simulink model "wrench_observer"  (R2018b)
settings: Solver=VariableStepAuto  StartTime=0.0  StopTime=0.75  RelTol=1e-3
InitFcn:
  | %x_k1 = 0.00001*ones(36,1); % initialisation with initial state uncertainity
  | %P_k1 = 0.00001*ones(36); % initialisation with initial state uncertainity
values from neighbouring files (symbols this model uses):
  a_noise = 0    [parameter.m]
  alpha1 = pi/2    (= 1.57079632679)    [parameter.m]
  alpha2 = 0    [parameter.m]
  alpha3 = 0    [parameter.m]
  angular_noise = 0    [parameter.m]
  g = 9.81    [parameter.m]
  K_f_comm = 1    [parameter.m]
  K_I = [500*eye(3), zeros(3), zeros(3) ... (first row only)    [parameter.m]
  K_tau_comm = 1    [parameter.m]
  K_tau_man_comm = 1    [parameter.m]
  m = 3.9    [parameter.m]
  m_l1 = 0.3    [parameter.m]
  m_l2 = 0.35    [parameter.m]
  m_l3 = 0.35    [parameter.m]
  N_m = 1*diag([(p_noise/(3*noise_factor))^2 (p_noise/(3*noise_factor))^2 (p_noise/(3*noise_factor))^2 (a_noise/(3*noise_factor))^2 (a_noise/(3*noise_factor))^2 (a_noise/(3*noise_factor))^2 (angular_noise/(3*noise_factor))^2 (angular_noise/(3*noise_factor))^2 (angular_noise/(3*noise_factor))^2 (omega_noise/(3*noise_factor))^2 (omega_noise/(3*noise_factor))^2 (omega_noise/(3*noise_factor))^2 (theta_noise/( ...(+272 chars)    [parameter.m]
  N_p = diag(noise_factor_EKF)    [parameter.m]
  omega_dot_noise = 0    [parameter.m]
  omega_noise = 0    [parameter.m]
  p_L1_l1 = [p_L1_x_l1 p_L1_y_l1 p_L1_z_l1]'    [parameter.m]
  p_L2_l2 = [p_L2_x_l2 p_L2_y_l2 p_L2_z_l2]'    [parameter.m]
  p_L3_l3 = [p_L3_x_l3 p_L3_y_l3 p_L3_z_l3]'    [parameter.m]
  p_noise = 0    [parameter.m]
  R_B_L0 = [1 0 0;0 1 0; 0 0 1]    [parameter.m]
  T_delay = 0    [parameter.m]
  T_dis = 0.01    [parameter.m]
  theta_dot_dot_noise = 0    [parameter.m]
  theta_dot_noise = 0    [parameter.m]
  theta_noise = 0    [parameter.m]
  Ts = 1/250    (= 0.004)    [parameter.m]
  v_noise = 0    [parameter.m]
libraries: simulink x9, dspstat3 x2, dspinverses x1
(part 1 of 5)
settings Model: SimulationMode=accelerator  Creator=Marek  LastModifiedBy=Marek
settings OptimizationCC: EfficientMapNaN2IntZero=off
settings HardwareCC: TargetBitPerPointer=64  TargetBitPerSizeT=64  TargetBitPerPtrDiffT=64  TargetLongLongMode=on  TargetIntDivRoundTo=Zero  TargetEndianess=LittleEndian  TargetWordSize=64  TargetHWDeviceType=MATLAB Host  ProdEqTarget=off
settings CodeAppCC: MaxIdLength=128
settings GRTTargetCC: TargetLangStandard=C89/C90 (ANSI)  CombineOutputUpdateFcns=off  GRTInterface=on

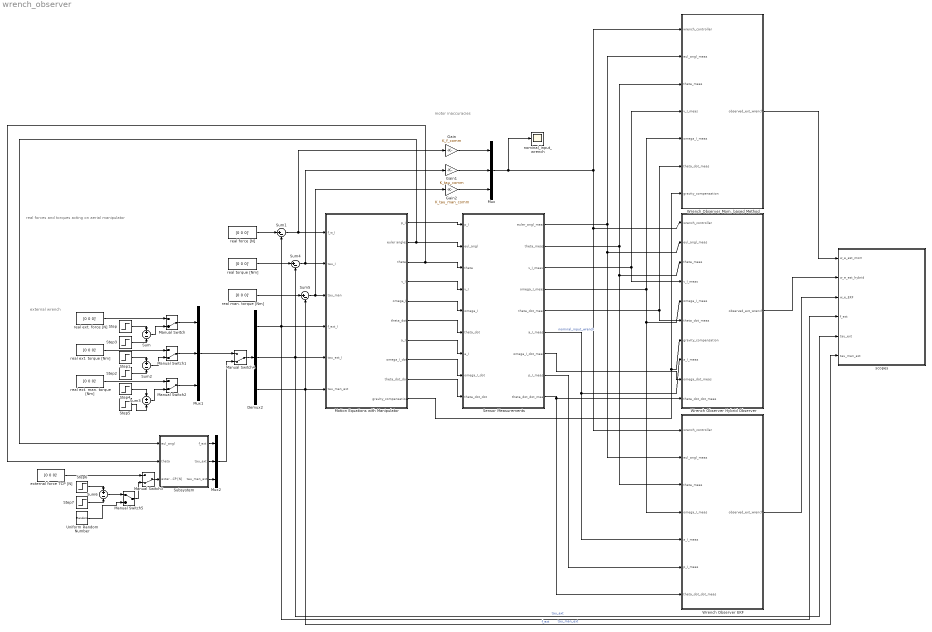
== system wrench_observer ==
  note: external wrench
  note: motor inaccuracies
  note: real forces and torques acting on aerial manipulator
  " external force TCP [N]" : Constant  Value=[0 0 0]'
  Demux2 : Demux  Outputs=3
  Gain : Gain  Gain=K_f_comm
  Gain1 : Gain  Gain=K_tau_comm
  Gain2 : Gain  Gain=K_tau_man_comm
  Manual Switch{,1..4} (5 alike) : ManualSwitch  CurrentSetting=0
  Manual Switch5 : ManualSwitch
  "Motion Equations with Manipulator " : Subsystem
  Mux : Mux  Inputs=3
  Mux1 : Mux  Inputs=3
  Mux2 : Mux  Inputs=3
  Sensor Measurements : Subsystem
  Step : Step  Time=0.2  Before=[0 0 0]'  After=[50 0 0]'  SampleTime=0
  Step1 : Step  Time=0.2  Before=[0 0 0]'  After=[0 100 0]'  SampleTime=0
  Step2 : Step  Time=0.7  Before=[0 0 0]'  After=[0 1 0]'  SampleTime=0
  Step3 : Step  Time=2.5  Before=[0 0 0]'  After=[50 0 0]'  SampleTime=0
  Step4 : Step  Time=0.2  Before=[0 0 0]'  After=[30 0 -45]'  SampleTime=0
  Step5 : Step  Time=0.7  Before=[0 0 0]'  After=[30 0 20]'  SampleTime=0
  Step6 : Step  Time=0.2  Before=[0 0 0]'  After=[50 0 -30]'  SampleTime=0
  Step7 : Step  Time=0.6  Before=[0 0 0]'  After=[50 0 -30]'  SampleTime=0
  Subsystem : Subsystem
  Sum{,2..3,6} (4 alike) : Sum  Inputs=+|-
  Sum1 : Sum  Inputs=|+-
  Sum4 : Sum  Inputs=|+-
  Sum5 : Sum  Inputs=|+-
  Uniform Random Number : UniformRandomNumber  Minimum=-50  Maximum=50  Seed=23  SampleTime=0.1
  Wrench Observer EKF : Subsystem
  Wrench Observer Hybrid Observer : Subsystem
  Wrench Observer Mom. based Method : Subsystem
  nominal_input_wrench : Scope
  real ext. force [N] : Constant  Value=[0 0 0]'
  real ext. man. torque [Nm] : Constant  Value=[0 0 0]'
  real ext. torque [Nm] : Constant  Value=[0 0 0]'
  real force [N] : Constant  Value=[0 0 0]'
  "real man. torque [Nm] " : Constant  Value=[0 0 0]'
  real torque [Nm] : Constant  Value=[0 0 0]'
  scopes : Subsystem
  wires:
  "Motion Equations with Manipulator "/1(p_I) -> Sensor Measurements/1(p_I)
  "Motion Equations with Manipulator "/2(euler angles) -> Subsystem/1(eul_angl), Sensor Measurements/2(eul_angl)
  "Motion Equations with Manipulator "/4(v_I) -> Sensor Measurements/4(v_I)
  "Motion Equations with Manipulator "/5(omega_I) -> Sensor Measurements/5(omega_I)
  "Motion Equations with Manipulator "/6(theta_dot) -> Sensor Measurements/6(theta_dot)
  "Motion Equations with Manipulator "/7(a_I) -> Sensor Measurements/7(a_I)
  "Motion Equations with Manipulator "/8(omega_I_dot) -> Sensor Measurements/8(omega_I_dot)
  "Motion Equations with Manipulator "/9(theta_dot_dot) -> Sensor Measurements/9(theta_dot_dot)
  Sum1/1 -> Gain/1, "Motion Equations with Manipulator "/1("f_w_I ")
  Sum5/1 -> Gain2/1, "Motion Equations with Manipulator "/3("tau_man ")
  Sum4/1 -> Gain1/1, "Motion Equations with Manipulator "/2(tau_I)
  Sensor Measurements/1(euler_angl_meas) -> Wrench Observer EKF/2(eul_angl_meas), Wrench Observer Hybrid Observer/2(eul_angl_meas), Wrench Observer Mom. based Method/2(eul_angl_meas)
  Sensor Measurements/2(theta_meas) -> Wrench Observer EKF/3(theta_meas), Wrench Observer Hybrid Observer/3(theta_meas), Wrench Observer Mom. based Method/3(theta_meas)
  Sensor Measurements/3(v_I_meas) -> Wrench Observer Hybrid Observer/4(v_I_meas), Wrench Observer Mom. based Method/4(v_I_meas)
  Sensor Measurements/4(omega_I_meas) -> Wrench Observer EKF/4(omega_I_meas), Wrench Observer Hybrid Observer/5(omega_I_meas), Wrench Observer Mom. based Method/5(omega_I_meas)
  Sensor Measurements/5(theta_dot_meas) -> Wrench Observer Hybrid Observer/6(theta_dot_meas), Wrench Observer Mom. based Method/6(theta_dot_meas)
  Sensor Measurements/6(a_I_meas) -> Wrench Observer Hybrid Observer/8(a_I_meas), Wrench Observer EKF/5(a_I_meas)
  Sensor Measurements/9(theta_dot_dot_meas) -> Wrench Observer Hybrid Observer/10(theta_dot_dot_meas), Wrench Observer EKF/7(theta_dot_dot_meas)
  Sensor Measurements/8(p_I_meas) -> Wrench Observer EKF/6(p_I_meas)
  Mux/1 -> nominal_input_wrench/1, Wrench Observer Mom. based Method/1(wrench_controller), Wrench Observer Hybrid Observer/1(wrench_controller), Wrench Observer EKF/1(wrench_controller)  "nominal_input_wrench"
  "Motion Equations with Manipulator "/10(gravity_compensation) -> Wrench Observer Hybrid Observer/7(gravity_compensation), Wrench Observer Mom. based Method/7(gravity_compensation)
  real ext. torque [Nm]/1 -> Manual Switch1/1
  real ext. man. torque [Nm]/1 -> Manual Switch2/1
  Step3/1 -> Sum/2
  Step/1 -> Sum/1
  Sum/1 -> Manual Switch/2
  Step2/1 -> Sum2/2
  Step1/1 -> Sum2/1
  Sum2/1 -> Manual Switch1/2
  Step5/1 -> Sum3/2
  Step4/1 -> Sum3/1
  Sum3/1 -> Manual Switch2/2
  real ext. force [N]/1 -> Manual Switch/1
  "Motion Equations with Manipulator "/3(theta) -> Sensor Measurements/3(theta), Subsystem/2(theta)
  Step6/1 -> Sum6/1
  Sum6/1 -> Manual Switch5/1
  Step7/1 -> Sum6/2
  Manual Switch3/1 -> Subsystem/3(external force TCP [N])
  Manual Switch/1 -> Mux1/1
  Manual Switch1/1 -> Mux1/2
  Manual Switch2/1 -> Mux1/3
  Demux2/1 -> scopes/4(f_ext), "Motion Equations with Manipulator "/4(f_ext_I), Sum1/2  "f_ext"
  Demux2/2 -> scopes/5(tau_ext), Sum4/2, "Motion Equations with Manipulator "/5(tau_ext_I)  "tau_ext"
  Demux2/3 -> scopes/6(tau_man_ext), Sum5/2, "Motion Equations with Manipulator "/6("tau_man_ext ")  "tau_man_ext"
  Mux1/1 -> Manual Switch4/1
  Subsystem/2(tau_ext) -> Mux2/2
  Subsystem/3(tau_man_ext) -> Mux2/3
  Subsystem/1(f_ext) -> Mux2/1
  Mux2/1 -> Manual Switch4/2
  Manual Switch4/1 -> Demux2/1
  Uniform Random Number/1 -> Manual Switch5/2
  Manual Switch5/1 -> Manual Switch3/2
  real force [N]/1 -> Sum1/1
  real torque [Nm]/1 -> Sum4/1
  "real man. torque [Nm] "/1 -> Sum5/1
  " external force TCP [N]"/1 -> Manual Switch3/1
  Gain/1 -> Mux/1
  Gain1/1 -> Mux/2
  Gain2/1 -> Mux/3
  Sensor Measurements/7(omega_I_dot_meas) -> Wrench Observer Hybrid Observer/9(omega_dot_meas)
  Wrench Observer Mom. based Method/1(observed_ext_wrench) -> scopes/1(w_e_est_mom)
  Wrench Observer Hybrid Observer/1(observed_ext_wrench) -> scopes/2(w_e_est_hybrid)
  Wrench Observer EKF/1(observed_ext_wrench) -> scopes/3(w_e_EKF)

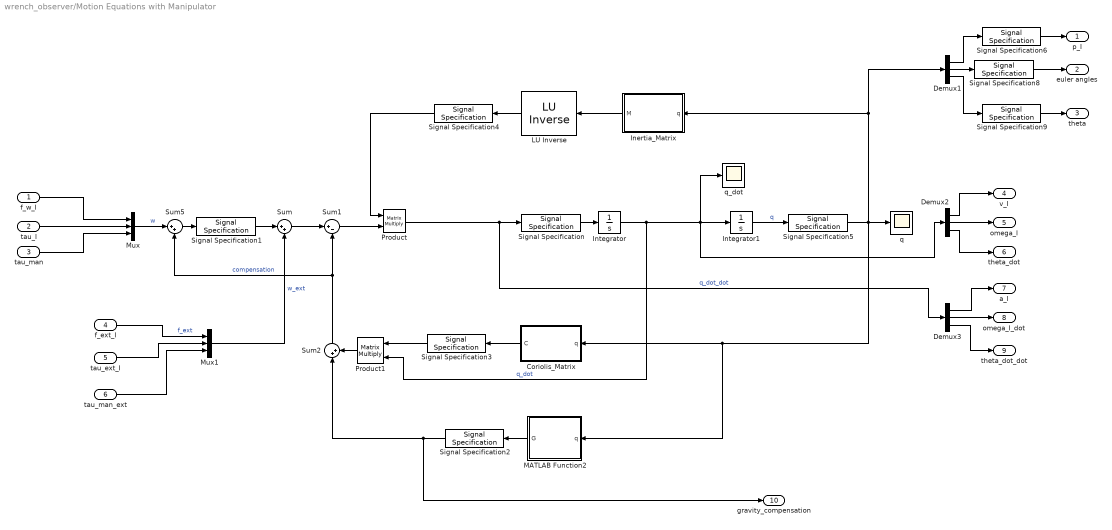
== system wrench_observer/Motion Equations with Manipulator  ==
  "f_w_I " : Inport
  tau_I : Inport  Port=2
  "tau_man " : Inport  Port=3
  f_ext_I : Inport  Port=4  PortDimensions=3
  tau_ext_I : Inport  Port=5  PortDimensions=3
  "tau_man_ext " : Inport  Port=6  PortDimensions=3
  " LU Inverse" : dspinverses/ LU Inverse
      settings: SourceProductName=DSP System Toolbox
  Coriolis_Matrix : Subsystem
  Demux1 : Demux  Outputs=3
  Demux2 : Demux  Outputs=3
  Demux3 : Demux  Outputs=3
  Inertia_Matrix : Subsystem
  Integrator : Integrator  InitialCondition=[0 0 0 0 0 0 0 0 0]'
  Integrator1 : Integrator  InitialCondition=[1 0.75 1 0.1 0.1 0.1 pi/3 pi/3 pi/3]'
  MATLAB Function2 : MATLAB Function  TreatAsAtomicUnit=on
  Mux : Mux  Inputs=3
  Mux1 : Mux  Inputs=3
  Product : Product  Multiplication=Matrix(*)  OutDataTypeStr=Inherit: Same as first input
  Product1 : Product  Multiplication=Matrix(*)
  Signal Specification{,1..2,5} (4 alike) : SignalSpecification  Dimensions=[9 1]
  Signal Specification3 : SignalSpecification  Dimensions=[9 9]
  Signal Specification4 : SignalSpecification  Dimensions=[9 9]
  Signal Specification6 : SignalSpecification  Dimensions=[3 1]
  Signal Specification8 : SignalSpecification  Dimensions=[3 1]
  Signal Specification9 : SignalSpecification  Dimensions=[3 1]
  Sum : Sum  Inputs=|++
  Sum1 : Sum  Inputs=|+-
  Sum2 : Sum  Inputs=|++
  Sum5 : Sum  Inputs=|++
  q : Scope
  q_dot : Scope
  p_I : Outport
  euler angles : Outport  Port=2
  theta : Outport  Port=3
  v_I : Outport  Port=4
  omega_I : Outport  Port=5
  theta_dot : Outport  Port=6
  a_I : Outport  Port=7
  omega_I_dot : Outport  Port=8
  theta_dot_dot : Outport  Port=9
  gravity_compensation : Outport  Port=10
  wires:
  "f_w_I "/1 -> Mux/1
  tau_I/1 -> Mux/2
  f_ext_I/1 -> Mux1/1  "f_ext"
  tau_ext_I/1 -> Mux1/2
  Mux/1 -> Sum5/1  "w"
  Sum/1 -> Sum1/1
  Sum2/1 -> Sum5/2, Sum1/2  "compensation"
  Integrator/1 -> q_dot/1, Demux2/1, Integrator1/1, Product1/2  "q_dot"
  Integrator1/1 -> Signal Specification5/1  "q"
  Sum1/1 -> Product/2
  Demux1/1 -> Signal Specification6/1
  Demux2/2 -> omega_I/1
  Demux1/3 -> Signal Specification9/1
  Demux2/1 -> v_I/1
  Demux2/3 -> theta_dot/1
  Demux3/1 -> a_I/1
  Demux3/2 -> omega_I_dot/1
  Demux3/3 -> theta_dot_dot/1
  Product1/1 -> Sum2/2
  "tau_man_ext "/1 -> Mux1/3
  "tau_man "/1 -> Mux/3
  Mux1/1 -> Sum/2  "w_ext"
  Signal Specification/1 -> Integrator/1
  Signal Specification1/1 -> Sum/1
  Signal Specification3/1 -> Product1/1
  " LU Inverse"/1 -> Signal Specification4/1
  Signal Specification4/1 -> Product/1
  Signal Specification5/1 -> Demux1/1, Inertia_Matrix/1(q), q/1, MATLAB Function2/1(q), Coriolis_Matrix/1(q)
  Demux1/2 -> Signal Specification8/1
  MATLAB Function2/1(G) -> Signal Specification2/1
  Inertia_Matrix/1(M) -> " LU Inverse"/1
  Coriolis_Matrix/1(C) -> Signal Specification3/1
  Signal Specification6/1 -> p_I/1
  Signal Specification8/1 -> euler angles/1
  Signal Specification9/1 -> theta/1
  Product/1 -> Demux3/1, Signal Specification/1  "q_dot_dot"
  Signal Specification2/1 -> gravity_compensation/1, Sum2/1
  Sum5/1 -> Signal Specification1/1

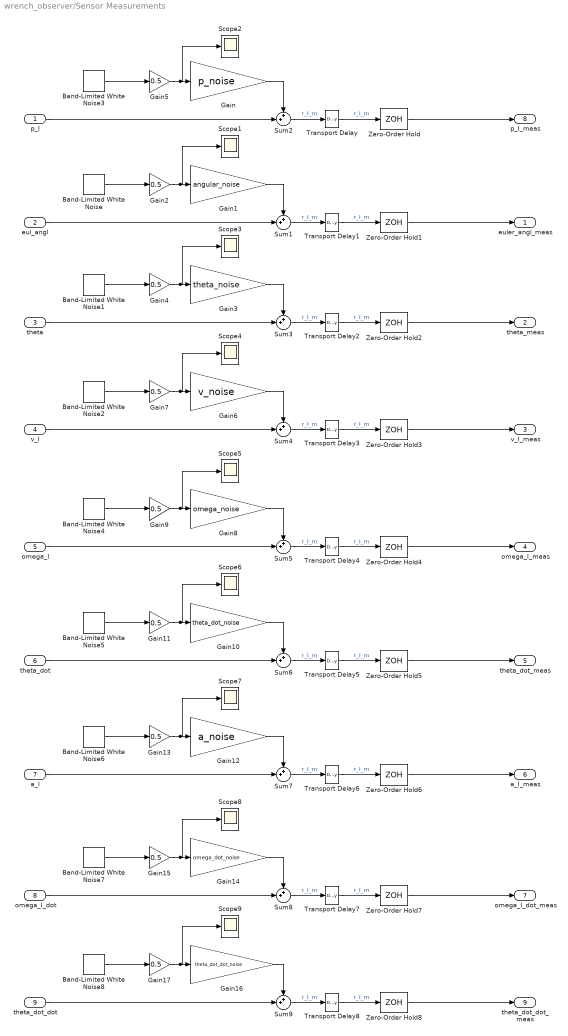
== system wrench_observer/Sensor Measurements ==
  p_I : Inport
  eul_angl : Inport  Port=2
  theta : Inport  Port=3
  v_I : Inport  Port=4
  omega_I : Inport  Port=5
  theta_dot : Inport  Port=6
  a_I : Inport  Port=7
  omega_I_dot : Inport  Port=8
  theta_dot_dot : Inport  Port=9
  Band-Limited White Noise : simulink/Sources/Band-Limited White Noise  Cov=noise_power  Ts=Ts  seed=[23341 2342 3453]'
  Band-Limited White Noise1 : simulink/Sources/Band-Limited White Noise  Cov=noise_power  Ts=Ts  seed=[23346 234 2345]'
  Band-Limited White Noise2 : simulink/Sources/Band-Limited White Noise  Cov=noise_power  Ts=Ts  seed=[233412 1234435 23]'
  Band-Limited White Noise3 : simulink/Sources/Band-Limited White Noise  Cov=noise_power  Ts=Ts  seed=[22352; 29655; 12541]  VectorParams1D=off
  Band-Limited White Noise4 : simulink/Sources/Band-Limited White Noise  Cov=noise_power  Ts=Ts  seed=[23341 34512 234345]'
  Band-Limited White Noise5 : simulink/Sources/Band-Limited White Noise  Cov=noise_power  Ts=Ts  seed=[23341 2345 231]'
  Band-Limited White Noise6 : simulink/Sources/Band-Limited White Noise  Cov=noise_power  Ts=Ts  seed=[235 3451 4352]'
  Band-Limited White Noise7 : simulink/Sources/Band-Limited White Noise  Cov=noise_power  Ts=Ts  seed=[3462 56735 1234]'
  Band-Limited White Noise8 : simulink/Sources/Band-Limited White Noise  Cov=noise_power  Ts=Ts  seed=[23341 2345 1234]'
  Gain : Gain  Gain=p_noise
  Gain1 : Gain  Gain=angular_noise
  Gain10 : Gain  Gain=theta_dot_noise
  Gain{2,4..5,7,9,11,13,15,17} (9 alike) : Gain  Gain=0.5
  Gain12 : Gain  Gain=a_noise
  Gain14 : Gain  Gain=omega_dot_noise
  Gain16 : Gain  Gain=theta_dot_dot_noise
  Gain3 : Gain  Gain=theta_noise
  Gain6 : Gain  Gain=v_noise
  Gain8 : Gain  Gain=omega_noise
  Scope{1..9} (9 alike) : Scope
  Sum{1..9} (9 alike) : Sum  Inputs=++|
  Transport Delay{,1..8} (9 alike) : TransportDelay  DelayTime=T_delay  InitialOutput=[0;0;0]
  Zero-Order Hold{,1..8} (9 alike) : ZeroOrderHold  SampleTime=0.02
  euler_angl_meas : Outport
  theta_meas : Outport  Port=2
  v_I_meas : Outport  Port=3
  omega_I_meas : Outport  Port=4
  theta_dot_meas : Outport  Port=5
  a_I_meas : Outport  Port=6
  omega_I_dot_meas : Outport  Port=7
  p_I_meas : Outport  Port=8
  theta_dot_dot_meas : Outport  Port=9
  wires:
  Gain5/1 -> Scope2/1, Gain/1
  Band-Limited White Noise3/1 -> Gain5/1
  Sum2/1 -> Transport Delay/1  "r_I_m"
  Gain/1 -> Sum2/1
  Transport Delay/1 -> Zero-Order Hold/1  "r_I_m"
  p_I/1 -> Sum2/2
  Zero-Order Hold/1 -> p_I_meas/1
  Transport Delay1/1 -> Zero-Order Hold1/1  "r_I_m"
  Sum1/1 -> Transport Delay1/1  "r_I_m"
  Band-Limited White Noise/1 -> Gain2/1
  Gain1/1 -> Sum1/1
  eul_angl/1 -> Sum1/2
  Gain2/1 -> Scope1/1, Gain1/1
  Zero-Order Hold1/1 -> euler_angl_meas/1
  Band-Limited White Noise1/1 -> Gain4/1
  Gain4/1 -> Scope3/1, Gain3/1
  Sum3/1 -> Transport Delay2/1  "r_I_m"
  Gain3/1 -> Sum3/1
  Zero-Order Hold2/1 -> theta_meas/1
  Transport Delay2/1 -> Zero-Order Hold2/1  "r_I_m"
  theta/1 -> Sum3/2
  Band-Limited White Noise2/1 -> Gain7/1
  Gain7/1 -> Scope4/1, Gain6/1
  Sum4/1 -> Transport Delay3/1  "r_I_m"
  Gain6/1 -> Sum4/1
  Zero-Order Hold3/1 -> v_I_meas/1
  Transport Delay3/1 -> Zero-Order Hold3/1  "r_I_m"
  v_I/1 -> Sum4/2
  Band-Limited White Noise4/1 -> Gain9/1
  Gain9/1 -> Scope5/1, Gain8/1
  Sum5/1 -> Transport Delay4/1  "r_I_m"
  Gain8/1 -> Sum5/1
  Zero-Order Hold4/1 -> omega_I_meas/1
  Transport Delay4/1 -> Zero-Order Hold4/1  "r_I_m"
  omega_I/1 -> Sum5/2
  Band-Limited White Noise5/1 -> Gain11/1
  Gain11/1 -> Scope6/1, Gain10/1
  Sum6/1 -> Transport Delay5/1  "r_I_m"
  Gain10/1 -> Sum6/1
  Zero-Order Hold5/1 -> theta_dot_meas/1
  Transport Delay5/1 -> Zero-Order Hold5/1  "r_I_m"
  theta_dot/1 -> Sum6/2
  Band-Limited White Noise6/1 -> Gain13/1
  Gain13/1 -> Scope7/1, Gain12/1
  Sum7/1 -> Transport Delay6/1  "r_I_m"
  Gain12/1 -> Sum7/1
  Zero-Order Hold6/1 -> a_I_meas/1
  Transport Delay6/1 -> Zero-Order Hold6/1  "r_I_m"
  a_I/1 -> Sum7/2
  Band-Limited White Noise7/1 -> Gain15/1
  Gain15/1 -> Scope8/1, Gain14/1
  Sum8/1 -> Transport Delay7/1  "r_I_m"
  Gain14/1 -> Sum8/1
  Zero-Order Hold7/1 -> omega_I_dot_meas/1
  Transport Delay7/1 -> Zero-Order Hold7/1  "r_I_m"
  omega_I_dot/1 -> Sum8/2
  Band-Limited White Noise8/1 -> Gain17/1
  Gain17/1 -> Scope9/1, Gain16/1
  Sum9/1 -> Transport Delay8/1  "r_I_m"
  Gain16/1 -> Sum9/1
  Zero-Order Hold8/1 -> theta_dot_dot_meas/1
  Transport Delay8/1 -> Zero-Order Hold8/1  "r_I_m"
  theta_dot_dot/1 -> Sum9/2

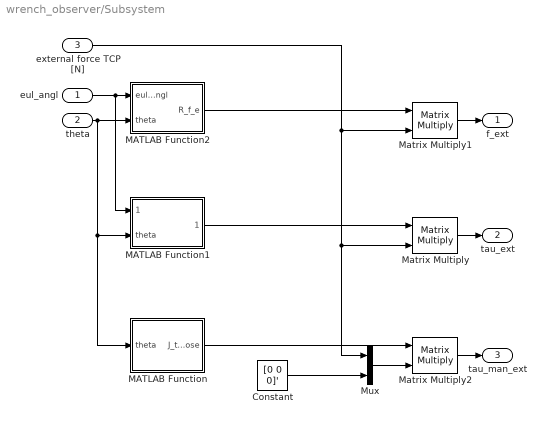
== system wrench_observer/Subsystem ==
  eul_angl : Inport
  theta : Inport  Port=2
  external force TCP [N] : Inport  Port=3
  Constant : Constant  Value=[0 0 0]'
  MATLAB Function : MATLAB Function  TreatAsAtomicUnit=on
  MATLAB Function1 : MATLAB Function  TreatAsAtomicUnit=on
  MATLAB Function2 : MATLAB Function  TreatAsAtomicUnit=on
  Matrix Multiply : Product  Multiplication=Matrix(*)
  Matrix Multiply1 : Product  Multiplication=Matrix(*)
  Matrix Multiply2 : Product  Multiplication=Matrix(*)
  Mux : Mux  Inputs=2
  f_ext : Outport
  tau_ext : Outport  Port=2
  tau_man_ext : Outport  Port=3
  wires:
  Matrix Multiply/1 -> tau_ext/1
  external force TCP [N]/1 -> Mux/1, Matrix Multiply/2, Matrix Multiply1/2
  Matrix Multiply2/1 -> tau_man_ext/1
  MATLAB Function/1(J_transpose) -> Matrix Multiply2/1
  Matrix Multiply1/1 -> f_ext/1
  MATLAB Function2/1(R_f_e) -> Matrix Multiply1/1
  MATLAB Function1/1(R_tau_e) -> Matrix Multiply/1
  eul_angl/1 -> MATLAB Function1/1(eul_angl), MATLAB Function2/1(eul_angl)
  theta/1 -> MATLAB Function1/2(theta), MATLAB Function/1(theta), MATLAB Function2/2(theta)
  Mux/1 -> Matrix Multiply2/2
  Constant/1 -> Mux/2

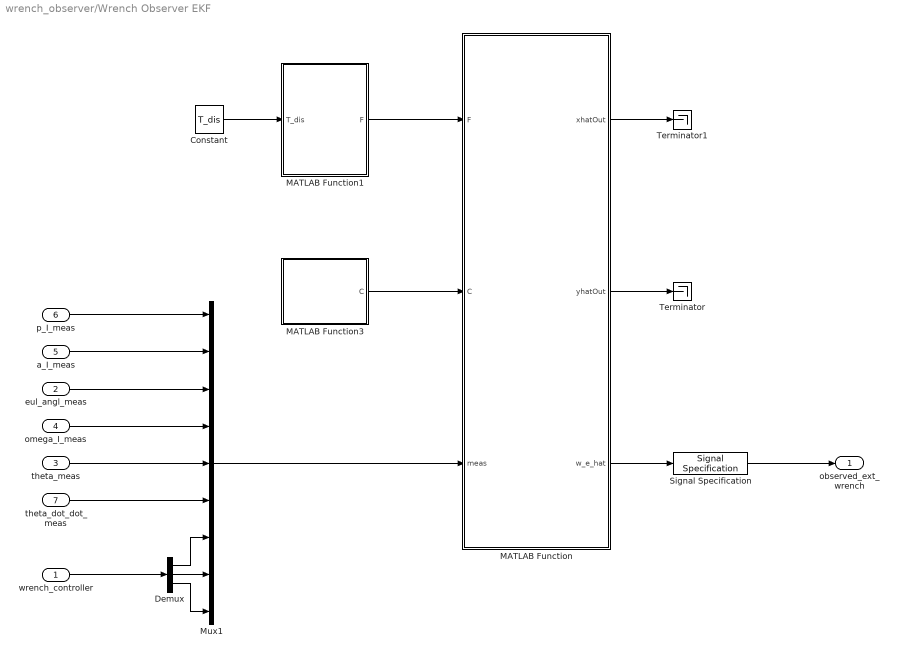
== system wrench_observer/Wrench Observer EKF ==
  wrench_controller : Inport
  eul_angl_meas : Inport  Port=2
  theta_meas : Inport  Port=3
  omega_I_meas : Inport  Port=4
  a_I_meas : Inport  Port=5
  p_I_meas : Inport  Port=6
  theta_dot_dot_meas : Inport  Port=7
  Constant : Constant  Value=T_dis
  Demux : Demux  Outputs=3
  MATLAB Function : MATLAB Function  InitFcn=|  TreatAsAtomicUnit=on
      | %x_k1 = [1 0.75 1 0 0 0 pi/4 pi/4 pi/4 0 0 0 pi/3 pi/3 pi/3 0 0 0 0 0 0 0 0 0 0 0 0 0 0 0 0 0 0 0 0 0]' 
      | %P_k1 = 0.0*ones(36); % initialisation with initial state uncertainity
      | %x_k_ = zeros(36,1);
      | %P_k_ = zeros(36);
      | %x_k = zeros(36,1);
      | %P_k = zeros(36);
  MATLAB Function1 : MATLAB Function  TreatAsAtomicUnit=on
  MATLAB Function3 : MATLAB Function  TreatAsAtomicUnit=on
  Mux1 : Mux  Inputs=9
  Signal Specification : SignalSpecification  Dimensions=[9 1]
  Terminator : Terminator
  Terminator1 : Terminator
  observed_ext_wrench : Outport
  wires:
  theta_dot_dot_meas/1 -> Mux1/6
  MATLAB Function/3(w_e_hat) -> Signal Specification/1
  Constant/1 -> MATLAB Function1/1(T_dis)
  MATLAB Function3/1(C) -> MATLAB Function/2(C)
  p_I_meas/1 -> Mux1/1
  a_I_meas/1 -> Mux1/2
  eul_angl_meas/1 -> Mux1/3
  omega_I_meas/1 -> Mux1/4
  theta_meas/1 -> Mux1/5
  MATLAB Function1/1(F) -> MATLAB Function/1(F)
  Demux/1 -> Mux1/7
  Demux/2 -> Mux1/8
  Demux/3 -> Mux1/9
  wrench_controller/1 -> Demux/1
  Mux1/1 -> MATLAB Function/3(meas)
  MATLAB Function/2(yhatOut) -> Terminator/1
  MATLAB Function/1(xhatOut) -> Terminator1/1
  Signal Specification/1 -> observed_ext_wrench/1

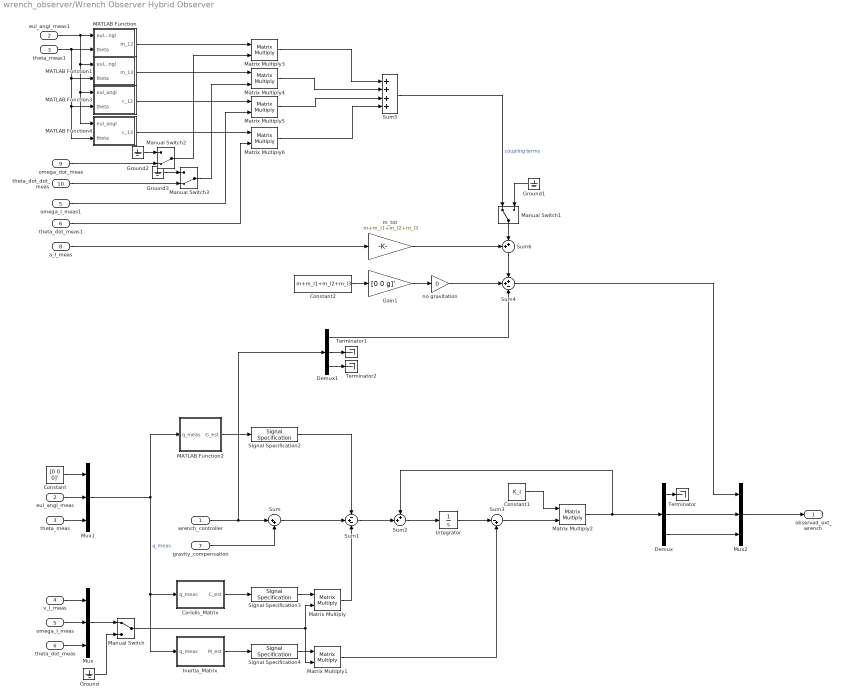
== system wrench_observer/Wrench Observer Hybrid Observer ==
  wrench_controller : Inport
  eul_angl_meas : Inport  Port=2
  theta_meas : Inport  Port=3
  v_I_meas : Inport  Port=4
  omega_I_meas : Inport  Port=5
  theta_dot_meas : Inport  Port=6
  gravity_compensation : Inport  Port=7
  a_I_meas : Inport  Port=8
  omega_dot_meas : Inport  Port=9
  theta_dot_dot_meas : Inport  Port=10
  Constant : Constant  Value=[0 0 0]'
  Constant1 : Constant  Value=K_I
  Constant2 : Constant  Value=m+m_l1+m_l2+m_l3
  Coriolis_Matrix : Subsystem
  Demux : Demux  Outputs=3
  Demux1 : Demux  Outputs=3
  Gain1 : Gain  Gain=[0 0 g]'
  Ground{,1..3} (4 alike) : Ground
  Inertia_Matrix : Subsystem
  Integrator : Integrator
  MATLAB Function : MATLAB Function  TreatAsAtomicUnit=on
  MATLAB Function1 : MATLAB Function  TreatAsAtomicUnit=on
  MATLAB Function2 : MATLAB Function  TreatAsAtomicUnit=on
  MATLAB Function3 : MATLAB Function  TreatAsAtomicUnit=on
  MATLAB Function4 : MATLAB Function  TreatAsAtomicUnit=on
  Manual Switch : ManualSwitch
  Manual Switch1 : ManualSwitch
  Manual Switch2 : ManualSwitch  CurrentSetting=0
  Manual Switch3 : ManualSwitch  CurrentSetting=0
  Matrix Multiply{,1..6} (7 alike) : Product  Multiplication=Matrix(*)
  Mux : Mux  Inputs=3
  Mux1 : Mux  Inputs=3
  Mux2 : Mux  Inputs=3
  Signal Specification2 : SignalSpecification  Dimensions=[9 1]
  Signal Specification3 : SignalSpecification  Dimensions=[9 9]
  Signal Specification4 : SignalSpecification  Dimensions=[9 9]
  Sum : Sum  Inputs=|++
  Sum1 : Sum  Inputs=-+-
  Sum2 : Sum  Inputs=++|
  Sum3 : Sum  Inputs=|-+
  Sum4 : Sum  Inputs=++-
  Sum5 : Sum  Inputs=++++
  Sum6 : Sum  Inputs=++|
  Terminator : Terminator
  Terminator1 : Terminator
  Terminator2 : Terminator
  eul_angl_meas1 : InportShadow  Port=2
  m_tot : Gain  Gain=m+m_l1+m_l2+m_l3
  no gravitation : Gain  Gain=0
  omega_I_meas1 : InportShadow  Port=5
  theta_dot_meas1 : InportShadow  Port=6
  theta_meas1 : InportShadow  Port=3
  observed_ext_wrench : Outport
  wires:
  wrench_controller/1 -> Demux1/1, Sum/1
  Signal Specification2/1 -> Sum1/1
  MATLAB Function2/1(G_est) -> Signal Specification2/1
  Sum/1 -> Sum1/2
  Sum1/1 -> Sum2/2
  Integrator/1 -> Sum3/1
  Inertia_Matrix/1(M_est) -> Signal Specification4/1
  Sum3/1 -> Matrix Multiply2/2
  Matrix Multiply2/1 -> Demux/1, Sum2/1
  Coriolis_Matrix/1(C_est) -> Signal Specification3/1
  omega_I_meas/1 -> Mux/2
  theta_dot_meas/1 -> Mux/3
  v_I_meas/1 -> Mux/1
  Signal Specification3/1 -> Matrix Multiply/1
  Manual Switch/1 -> Matrix Multiply/2, Matrix Multiply1/2
  Signal Specification4/1 -> Matrix Multiply1/1
  theta_meas/1 -> Mux1/3
  eul_angl_meas/1 -> Mux1/2
  Constant/1 -> Mux1/1
  Mux1/1 -> MATLAB Function2/1(q_meas), Inertia_Matrix/1(q_meas), Coriolis_Matrix/1(q_meas)  "q_meas"
  Matrix Multiply/1 -> Sum1/3
  Matrix Multiply1/1 -> Sum3/2
  Constant1/1 -> Matrix Multiply2/1
  gravity_compensation/1 -> Sum/2
  Demux/2 -> Mux2/2
  Demux/3 -> Mux2/3
  Mux2/1 -> observed_ext_wrench/1
  Demux/1 -> Terminator/1
  a_I_meas/1 -> m_tot/1
  Constant2/1 -> Gain1/1
  Sum4/1 -> Mux2/1
  Mux/1 -> Manual Switch/1
  Ground/1 -> Manual Switch/2
  Demux1/1 -> Sum4/3
  Demux1/2 -> Terminator1/1
  Demux1/3 -> Terminator2/1
  Sum2/1 -> Integrator/1
  Gain1/1 -> no gravitation/1
  no gravitation/1 -> Sum4/2
  eul_angl_meas1/1 -> MATLAB Function1/1(eul_angl), MATLAB Function3/1(eul_angl), MATLAB Function4/1(eul_angl), MATLAB Function/1(eul_angl)
  theta_meas1/1 -> MATLAB Function1/2(theta), MATLAB Function3/2(theta), MATLAB Function4/2(theta), MATLAB Function/2(theta)
  MATLAB Function/1(m_12) -> Matrix Multiply3/1
  MATLAB Function1/1(m_13) -> Matrix Multiply4/1
  MATLAB Function3/1(c_12) -> Matrix Multiply5/1
  MATLAB Function4/1(c_13) -> Matrix Multiply6/1
  omega_I_meas1/1 -> Matrix Multiply5/2
  theta_dot_meas1/1 -> Matrix Multiply6/2
  Matrix Multiply3/1 -> Sum5/1
  Matrix Multiply4/1 -> Sum5/2
  Matrix Multiply5/1 -> Sum5/3
  Matrix Multiply6/1 -> Sum5/4
  m_tot/1 -> Sum6/1
  Sum5/1 -> Manual Switch1/1  "coupling terms"
  Sum6/1 -> Sum4/1
  Manual Switch1/1 -> Sum6/2
  Ground1/1 -> Manual Switch1/2
  omega_dot_meas/1 -> Manual Switch2/2
  theta_dot_dot_meas/1 -> Manual Switch3/2
  Manual Switch3/1 -> Matrix Multiply4/2
  Manual Switch2/1 -> Matrix Multiply3/2
  Ground2/1 -> Manual Switch2/1
  Ground3/1 -> Manual Switch3/1

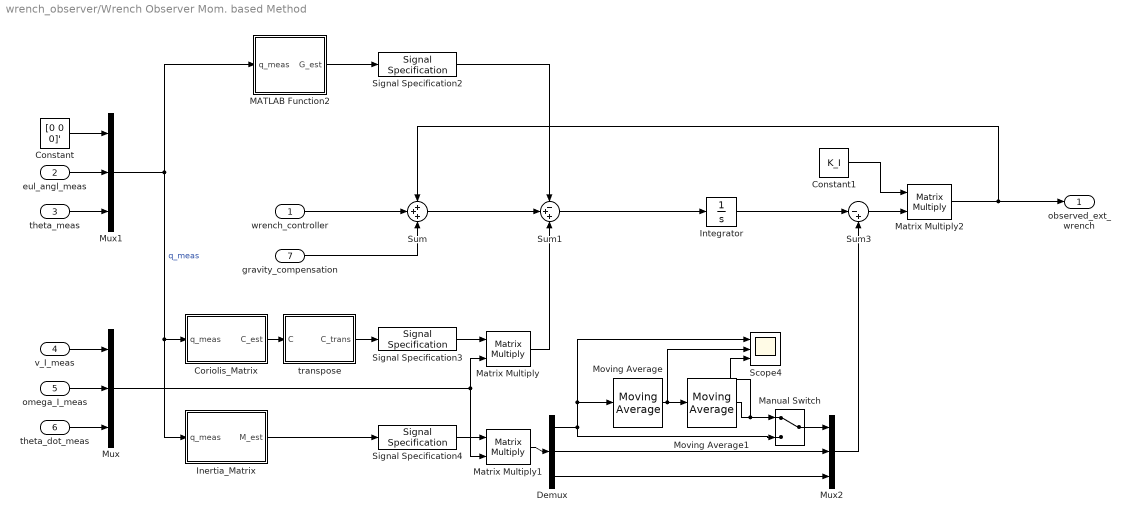
== system wrench_observer/Wrench Observer Mom. based Method ==
  wrench_controller : Inport
  eul_angl_meas : Inport  Port=2
  theta_meas : Inport  Port=3
  v_I_meas : Inport  Port=4
  omega_I_meas : Inport  Port=5
  theta_dot_meas : Inport  Port=6
  gravity_compensation : Inport  Port=7
  Constant : Constant  Value=[0 0 0]'
  Constant1 : Constant  Value=K_I
  Coriolis_Matrix : Subsystem
  Demux : Demux  Outputs=3
  Inertia_Matrix : Subsystem
  Integrator : Integrator
  MATLAB Function2 : MATLAB Function  TreatAsAtomicUnit=on
  Manual Switch : ManualSwitch
  Matrix Multiply : Product  Multiplication=Matrix(*)
  Matrix Multiply1 : Product  Multiplication=Matrix(*)
  Matrix Multiply2 : Product  Multiplication=Matrix(*)
  Moving Average : dspstat3/Moving Average  Method=Sliding window  ForgettingFactorPort=off  SpecifyWindowLength=on  WindowLength=10  ForgettingFactor=0.9  SimulateUsing=Interpreted execution
  Moving Average1 : dspstat3/Moving Average  Method=Sliding window  ForgettingFactorPort=off  SpecifyWindowLength=on  WindowLength=10  ForgettingFactor=0.9  SimulateUsing=Interpreted execution
  Mux : Mux  Inputs=3
  Mux1 : Mux  Inputs=3
  Mux2 : Mux  Inputs=3
  Scope4 : Scope  NumInputPorts=3
  Signal Specification2 : SignalSpecification  Dimensions=[9 1]
  Signal Specification3 : SignalSpecification  Dimensions=[9 9]
  Signal Specification4 : SignalSpecification  Dimensions=[9 9]
  Sum : Sum  Inputs=+++
  Sum1 : Sum  Inputs=-++
  Sum3 : Sum  Inputs=|-+
  transpose : MATLAB Function  TreatAsAtomicUnit=on
  observed_ext_wrench : Outport
  wires:
  wrench_controller/1 -> Sum/2
  Signal Specification2/1 -> Sum1/1
  MATLAB Function2/1(G_est) -> Signal Specification2/1
  Sum/1 -> Sum1/2
  Sum1/1 -> Integrator/1
  Integrator/1 -> Sum3/1
  Inertia_Matrix/1(M_est) -> Signal Specification4/1
  Sum3/1 -> Matrix Multiply2/2
  Matrix Multiply2/1 -> observed_ext_wrench/1, Sum/1
  omega_I_meas/1 -> Mux/2
  theta_dot_meas/1 -> Mux/3
  Signal Specification3/1 -> Matrix Multiply/1
  Mux/1 -> Matrix Multiply1/2, Matrix Multiply/2
  Signal Specification4/1 -> Matrix Multiply1/1
  theta_meas/1 -> Mux1/3
  eul_angl_meas/1 -> Mux1/2
  Constant/1 -> Mux1/1
  Mux1/1 -> MATLAB Function2/1(q_meas), Inertia_Matrix/1(q_meas), Coriolis_Matrix/1(q_meas)  "q_meas"
  Matrix Multiply/1 -> Sum1/3
  Constant1/1 -> Matrix Multiply2/1
  gravity_compensation/1 -> Sum/3
  v_I_meas/1 -> Mux/1
  Demux/3 -> Mux2/3
  Matrix Multiply1/1 -> Demux/1
  Demux/2 -> Mux2/2
  Mux2/1 -> Sum3/2
  Demux/1 -> Manual Switch/2, Scope4/1, Moving Average/1
  Moving Average/1 -> Scope4/2, Moving Average1/1
  Moving Average1/1 -> Scope4/3, Manual Switch/1
  Coriolis_Matrix/1(C_est) -> transpose/1(C)
  transpose/1(C_trans) -> Signal Specification3/1
  Manual Switch/1 -> Mux2/1

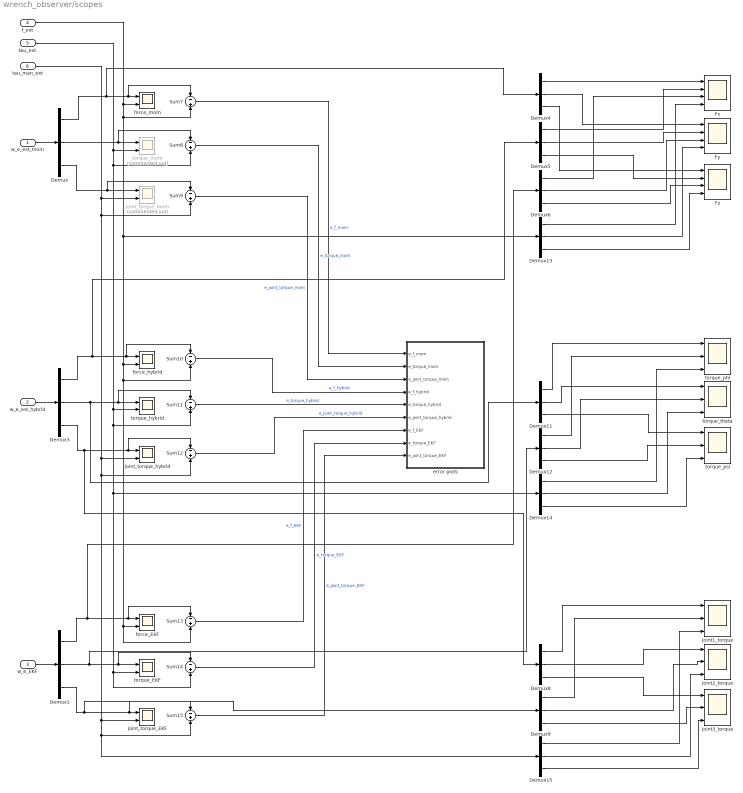
== system wrench_observer/scopes ==
  w_e_est_mom : Inport
  w_e_est_hybrid : Inport  Port=2
  w_e_EKF : Inport  Port=3
  f_ext : Inport  Port=4
  tau_ext : Inport  Port=5
  tau_man_ext : Inport  Port=6
  Demux{,1,3..6,8..9,11..15} (13 alike) : Demux  Outputs=3
  Fx : Scope  NumInputPorts=4
  Fy : Scope  NumInputPorts=4
  Fz : Scope  NumInputPorts=4
  Sum{7..15} (9 alike) : Sum  Inputs=-|+
  error plots : Subsystem
  force_EKF : Scope  NumInputPorts=2
  force_hybrid : Scope  NumInputPorts=2
  force_mom : Scope  NumInputPorts=2
  joint1_torque : Scope  NumInputPorts=3
  joint2_torque : Scope  NumInputPorts=3
  joint3_torque : Scope  NumInputPorts=3
  joint_torque_EKF : Scope  NumInputPorts=2
  joint_torque_hybrid : Scope  NumInputPorts=2
  joint_torque_mom : Scope  Commented=on  NumInputPorts=2
  torque_EKF : Scope  NumInputPorts=2
  torque_hybrid : Scope  NumInputPorts=2
  torque_mom : Scope  Commented=on  NumInputPorts=2
  torque_phi : Scope  NumInputPorts=3
  torque_psi : Scope  NumInputPorts=3
  torque_theta : Scope  NumInputPorts=3
  wires:
  Sum9/1 -> error plots/3(e_joint_torque_mom)  "e_joint_torque_mom"
  Demux3/3 -> Demux8/1, Sum12/1, joint_torque_hybrid/1
  Demux6/2 -> Fy/3
  tau_man_ext/1 -> Demux15/1, Sum15/2, joint_torque_EKF/2, Sum12/2, joint_torque_hybrid/2, Sum9/2, joint_torque_mom/2
  Demux/2 -> torque_mom/1, Sum8/1
  Demux3/1 -> Demux5/1, Sum10/1, force_hybrid/1
  Demux/1 -> Demux4/1, Sum7/1, force_mom/1
  f_ext/1 -> Sum13/2, force_EKF/2, Sum10/2, force_hybrid/2, Demux13/1, Sum7/2, force_mom/2
  tau_ext/1 -> Sum14/2, torque_EKF/2, Demux14/1, Sum11/2, torque_hybrid/2, Sum8/2, torque_mom/2
  Sum10/1 -> error plots/4(e_f_hybrid)  "e_f_hybrid"
  Demux12/1 -> torque_phi/2
  Demux/3 -> joint_torque_mom/1, Sum9/1
  Demux3/2 -> Demux11/1, Sum11/1, torque_hybrid/1
  Demux14/2 -> torque_theta/3
  Demux1/2 -> Demux12/1, Sum14/1, torque_EKF/1
  Demux1/1 -> Demux6/1, Sum13/1, force_EKF/1
  Demux6/1 -> Fx/3
  Demux4/1 -> Fx/1
  Demux5/1 -> Fx/2
  Demux8/1 -> joint1_torque/1
  Demux6/3 -> Fz/3
  Sum15/1 -> error plots/9(e_joint_torque_EKF)  "e_joint_torque_EKF"
  Demux4/2 -> Fy/1
  Demux1/3 -> Demux9/1, Sum15/1, joint_torque_EKF/1
  Demux15/2 -> joint2_torque/3
  Demux5/3 -> Fz/2
  Demux9/1 -> joint1_torque/2
  Demux4/3 -> Fz/1
  Demux11/2 -> torque_theta/1
  Sum7/1 -> error plots/1(e_f_mom)  "e_f_mom"
  Demux15/1 -> joint1_torque/3
  Demux5/2 -> Fy/2
  w_e_est_mom/1 -> Demux/1
  Demux13/2 -> Fy/4
  Sum14/1 -> error plots/8(e_torque_EKF)  "e_torque_EKF"
  Sum12/1 -> error plots/6(e_joint_torque_hybrid)  "e_joint_torque_hybrid"
  Demux13/3 -> Fz/4
  Demux12/2 -> torque_theta/2
  Demux14/1 -> torque_phi/3
  Demux8/3 -> joint3_torque/1
  Demux11/1 -> torque_phi/1
  Demux11/3 -> torque_psi/1
  Demux15/3 -> joint3_torque/3
  Demux9/2 -> joint2_torque/2
  Sum11/1 -> error plots/5(e_torque_hybrid)  "e_torque_hybrid"
  Sum13/1 -> error plots/7(e_f_EKF)  "e_f_EKF"
  Demux8/2 -> joint2_torque/1
  Demux9/3 -> joint3_torque/2
  Demux13/1 -> Fx/4
  Demux14/3 -> torque_psi/3
  Demux12/3 -> torque_psi/2
  Sum8/1 -> error plots/2(e_torque_mom)  "e_torque_mom"
  w_e_EKF/1 -> Demux1/1
  w_e_est_hybrid/1 -> Demux3/1

== system wrench_observer/Motion Equations with Manipulator /Coriolis_Matrix ==
  q : Inport
  Coriolis_Matrix_simplified : Subsystem
  Demux : Demux  Outputs=9
  Terminator : Terminator
  Terminator1 : Terminator
  Terminator2 : Terminator
  C : Outport
  wires:
  Demux/1 -> Terminator/1
  Demux/2 -> Terminator1/1
  Demux/6 -> Coriolis_Matrix_simplified/3(psi)
  Demux/5 -> Coriolis_Matrix_simplified/2(the)
  Demux/7 -> Coriolis_Matrix_simplified/4(theta1)
  Demux/8 -> Coriolis_Matrix_simplified/5(theta2)
  Demux/4 -> Coriolis_Matrix_simplified/1(phi)
  Demux/9 -> Coriolis_Matrix_simplified/6(theta3)
  Demux/3 -> Terminator2/1
  Coriolis_Matrix_simplified/1(C) -> C/1
  q/1 -> Demux/1

== system wrench_observer/Motion Equations with Manipulator /Inertia_Matrix ==
  q : Inport
  Demux4 : Demux  Outputs=9
  S-Function Builder : S-Function  InitFcn=try, set_param(gcb,'FunctionName','Inertia_Matrix_simplified'), end  FunctionName=Inertia_Matrix_simplified  SFunctionModules=Inertia_Matrix_simplified_wrapper Inertia_Matrix Inertia_Matrix_initialize Inertia_Matrix_terminate rt_nonfinite rtGetInf rtGetNaN  SFunctionDeploymentMode=off  EnableBusSupport=off  mask(S-Function Builder){}
      mask help: Simulink:masks:SFunctionBuilder_MD
      mask init:
      | val = [[.9  0.75 0.75 1 1 .9 .9 1]',[1 1 0.75 0.75 .9 .9 1 .9]'];try , sys = get_param(gcb,'SfunBuilderFcnName');if isempty(sys), sys = get_param(gcb,'FunctionName'); end,catch, sys = get_param(gcb,'FunctionName'); end
      settings: CopyFcn=set_param(gcbh,'LinkStatus','none')  PreSaveFcn=try, set_param(gcb,'FunctionName','Inertia_Matrix_simplified'), end  OpenFcn=sfunctionwizard(gcbh)
      mask Display: plot(val(:,1),val(:,2)),disp(sys), port_label('input',1,'phi'), port_label('input',2,'the'), port_label('input',3,'psi'), port_label('input',4,'theta1'), port_label('input',5,'theta2'), port_label('input',6,'theta3'), port_label('output',1,'M')
  Terminator3 : Terminator
  Terminator4 : Terminator
  Terminator5 : Terminator
  M : Outport
  wires:
  Demux4/4 -> S-Function Builder/1
  Demux4/1 -> Terminator3/1
  Demux4/7 -> S-Function Builder/4
  Demux4/5 -> S-Function Builder/2
  Demux4/9 -> S-Function Builder/6
  Demux4/6 -> S-Function Builder/3
  q/1 -> Demux4/1
  Demux4/2 -> Terminator4/1
  Demux4/3 -> Terminator5/1
  Demux4/8 -> S-Function Builder/5
  S-Function Builder/1 -> M/1

== system wrench_observer/Wrench Observer Hybrid Observer/Coriolis_Matrix ==
  q_meas : Inport
  Coriolis_Matrix_simplified : Subsystem
  Demux : Demux  Outputs=9
  Terminator : Terminator
  Terminator1 : Terminator
  Terminator2 : Terminator
  C_est : Outport
  wires:
  Demux/1 -> Terminator/1
  Demux/2 -> Terminator1/1
  Demux/6 -> Coriolis_Matrix_simplified/3(psi)
  Demux/5 -> Coriolis_Matrix_simplified/2(the)
  Demux/7 -> Coriolis_Matrix_simplified/4(theta1)
  Demux/8 -> Coriolis_Matrix_simplified/5(theta2)
  Demux/4 -> Coriolis_Matrix_simplified/1(phi)
  Demux/9 -> Coriolis_Matrix_simplified/6(theta3)
  Demux/3 -> Terminator2/1
  Coriolis_Matrix_simplified/1(C) -> C_est/1
  q_meas/1 -> Demux/1

== system wrench_observer/Wrench Observer Hybrid Observer/Inertia_Matrix ==
  q_meas : Inport
  Demux4 : Demux  Outputs=9
  S-Function Builder : S-Function  InitFcn=try, set_param(gcb,'FunctionName','Inertia_Matrix_simplified'), end  FunctionName=Inertia_Matrix_simplified  SFunctionModules=Inertia_Matrix_simplified_wrapper Inertia_Matrix Inertia_Matrix_initialize Inertia_Matrix_terminate rt_nonfinite rtGetInf rtGetNaN  SFunctionDeploymentMode=off  EnableBusSupport=off  mask(S-Function Builder){}
      mask help: Simulink:masks:SFunctionBuilder_MD
      mask init: same as wrench_observer/Motion Equations with Manipulator /Inertia_Matrix/S-Function Builder
      settings: CopyFcn=set_param(gcbh,'LinkStatus','none')  PreSaveFcn=try, set_param(gcb,'FunctionName','Inertia_Matrix_simplified'), end  OpenFcn=sfunctionwizard(gcbh)
      mask Display: plot(val(:,1),val(:,2)),disp(sys), port_label('input',1,'phi'), port_label('input',2,'the'), port_label('input',3,'psi'), port_label('input',4,'theta1'), port_label('input',5,'theta2'), port_label('input',6,'theta3'), port_label('output',1,'M')
  Terminator3 : Terminator
  Terminator4 : Terminator
  Terminator5 : Terminator
  M_est : Outport
  wires:
  Demux4/4 -> S-Function Builder/1
  Demux4/1 -> Terminator3/1
  Demux4/7 -> S-Function Builder/4
  Demux4/5 -> S-Function Builder/2
  Demux4/9 -> S-Function Builder/6
  Demux4/6 -> S-Function Builder/3
  q_meas/1 -> Demux4/1
  Demux4/2 -> Terminator4/1
  Demux4/3 -> Terminator5/1
  Demux4/8 -> S-Function Builder/5
  S-Function Builder/1 -> M_est/1

== system wrench_observer/Wrench Observer Mom. based Method/Coriolis_Matrix ==
  q_meas : Inport
  Coriolis_Matrix_simplified : Subsystem
  Demux : Demux  Outputs=9
  Terminator : Terminator
  Terminator1 : Terminator
  Terminator2 : Terminator
  C_est : Outport
  wires:
  Demux/1 -> Terminator/1
  Demux/2 -> Terminator1/1
  Demux/6 -> Coriolis_Matrix_simplified/3(psi)
  Demux/5 -> Coriolis_Matrix_simplified/2(the)
  Demux/7 -> Coriolis_Matrix_simplified/4(theta1)
  Demux/8 -> Coriolis_Matrix_simplified/5(theta2)
  Demux/4 -> Coriolis_Matrix_simplified/1(phi)
  Demux/9 -> Coriolis_Matrix_simplified/6(theta3)
  Demux/3 -> Terminator2/1
  Coriolis_Matrix_simplified/1(C) -> C_est/1
  q_meas/1 -> Demux/1

== system wrench_observer/Wrench Observer Mom. based Method/Inertia_Matrix ==
  q_meas : Inport
  Demux4 : Demux  Outputs=9
  S-Function Builder : S-Function  InitFcn=try, set_param(gcb,'FunctionName','Inertia_Matrix_simplified'), end  FunctionName=Inertia_Matrix_simplified  SFunctionModules=Inertia_Matrix_simplified_wrapper Inertia_Matrix Inertia_Matrix_initialize Inertia_Matrix_terminate rt_nonfinite rtGetInf rtGetNaN  SFunctionDeploymentMode=off  EnableBusSupport=off  mask(S-Function Builder){}
      mask help: Simulink:masks:SFunctionBuilder_MD
      mask init: same as wrench_observer/Motion Equations with Manipulator /Inertia_Matrix/S-Function Builder
      settings: CopyFcn=set_param(gcbh,'LinkStatus','none')  PreSaveFcn=try, set_param(gcb,'FunctionName','Inertia_Matrix_simplified'), end  OpenFcn=sfunctionwizard(gcbh)
      mask Display: plot(val(:,1),val(:,2)),disp(sys), port_label('input',1,'phi'), port_label('input',2,'the'), port_label('input',3,'psi'), port_label('input',4,'theta1'), port_label('input',5,'theta2'), port_label('input',6,'theta3'), port_label('output',1,'M')
  Terminator3 : Terminator
  Terminator4 : Terminator
  Terminator5 : Terminator
  M_est : Outport
  wires:
  Demux4/4 -> S-Function Builder/1
  Demux4/1 -> Terminator3/1
  Demux4/7 -> S-Function Builder/4
  Demux4/5 -> S-Function Builder/2
  Demux4/9 -> S-Function Builder/6
  Demux4/6 -> S-Function Builder/3
  q_meas/1 -> Demux4/1
  Demux4/2 -> Terminator4/1
  Demux4/3 -> Terminator5/1
  Demux4/8 -> S-Function Builder/5
  S-Function Builder/1 -> M_est/1

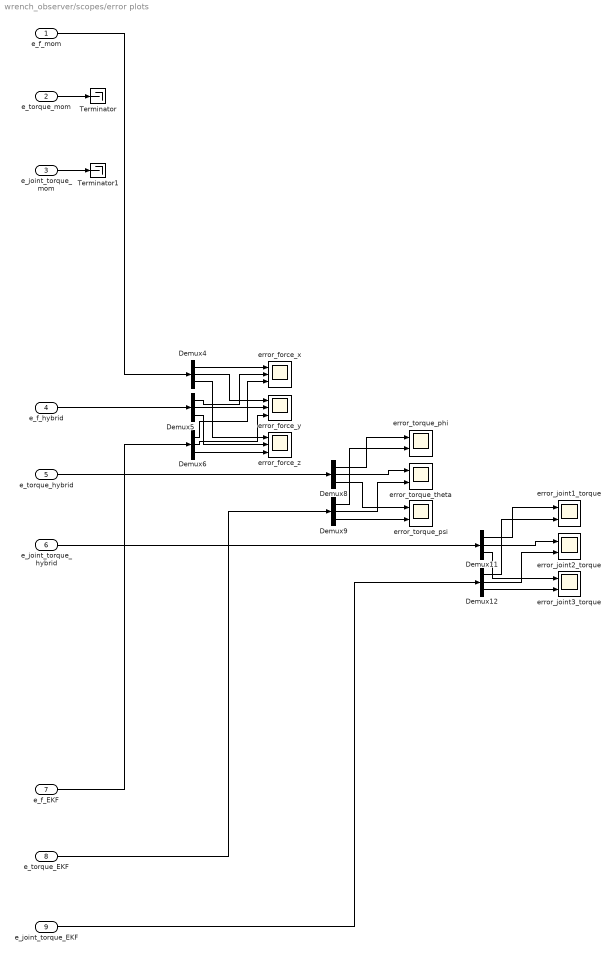
== system wrench_observer/scopes/error plots ==
  e_f_mom : Inport
  e_torque_mom : Inport  Port=2
  e_joint_torque_mom : Inport  Port=3
  e_f_hybrid : Inport  Port=4
  e_torque_hybrid : Inport  Port=5
  e_joint_torque_hybrid : Inport  Port=6
  e_f_EKF : Inport  Port=7
  e_torque_EKF : Inport  Port=8
  e_joint_torque_EKF : Inport  Port=9
  Demux{4..6,8..9,11..12} (7 alike) : Demux  Outputs=3
  Terminator : Terminator
  Terminator1 : Terminator
  error_force_x : Scope  NumInputPorts=3
  error_force_y : Scope  NumInputPorts=3
  error_force_z : Scope  NumInputPorts=3
  error_joint1_torque : Scope  NumInputPorts=2
  error_joint2_torque : Scope  NumInputPorts=2
  error_joint3_torque : Scope  NumInputPorts=2
  error_torque_phi : Scope  NumInputPorts=2
  error_torque_psi : Scope  NumInputPorts=2
  error_torque_theta : Scope  NumInputPorts=2
  wires:
  Demux6/3 -> error_force_z/3
  e_f_EKF/1 -> Demux6/1
  Demux4/1 -> error_force_x/1
  Demux5/2 -> error_force_y/2
  e_f_hybrid/1 -> Demux5/1
  e_torque_EKF/1 -> Demux9/1
  e_joint_torque_EKF/1 -> Demux12/1
  Demux5/1 -> error_force_x/2
  Demux4/2 -> error_force_y/1
  Demux6/2 -> error_force_y/3
  Demux5/3 -> error_force_z/2
  Demux4/3 -> error_force_z/1
  Demux6/1 -> error_force_x/3
  e_joint_torque_hybrid/1 -> Demux11/1
  e_torque_hybrid/1 -> Demux8/1
  e_f_mom/1 -> Demux4/1
  Demux8/1 -> error_torque_phi/1
  Demux8/2 -> error_torque_theta/1
  Demux8/3 -> error_torque_psi/1
  Demux9/1 -> error_torque_phi/2
  Demux9/2 -> error_torque_theta/2
  Demux9/3 -> error_torque_psi/2
  Demux11/1 -> error_joint1_torque/1
  Demux11/2 -> error_joint2_torque/1
  Demux12/1 -> error_joint1_torque/2
  Demux11/3 -> error_joint3_torque/1
  Demux12/2 -> error_joint2_torque/2
  Demux12/3 -> error_joint3_torque/2
  e_torque_mom/1 -> Terminator/1
  e_joint_torque_mom/1 -> Terminator1/1

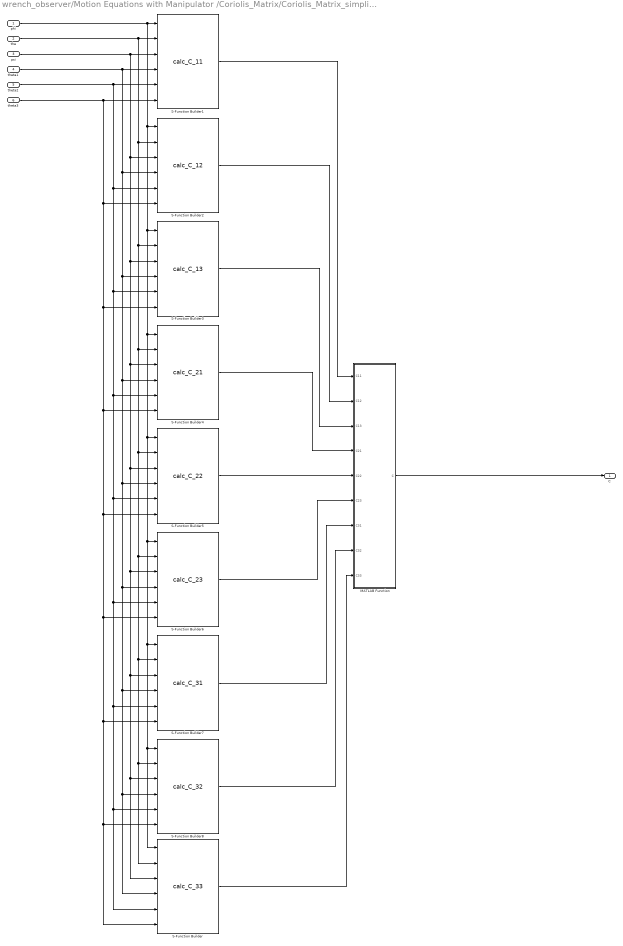
== system wrench_observer/Motion Equations with Manipulator /Coriolis_Matrix/Coriolis_Matrix_simplified ==
  phi : Inport
  the : Inport  Port=2
  psi : Inport  Port=3
  theta1 : Inport  Port=4
  theta2 : Inport  Port=5
  theta3 : Inport  Port=6
  MATLAB Function : MATLAB Function  TreatAsAtomicUnit=on
  S-Function Builder : S-Function  InitFcn=try, set_param(gcb,'FunctionName','calc_C_33'), end  FunctionName=calc_C_33  SFunctionModules=calc_C_33_wrapper C_num_simp_33 C_num_simp_33_initialize C_num_simp_33_terminate rt_nonfinite rtGetInf rtGetNaN  SFunctionDeploymentMode=off  EnableBusSupport=off  mask(S-Function Builder){}
      mask help: Simulink:masks:SFunctionBuilder_MD
      mask init: same as wrench_observer/Motion Equations with Manipulator /Inertia_Matrix/S-Function Builder
      settings: CopyFcn=set_param(gcbh,'LinkStatus','none')  PreSaveFcn=try, set_param(gcb,'FunctionName','calc_C_33'), end  OpenFcn=sfunctionwizard(gcbh)
      mask Display: plot(val(:,1),val(:,2)),disp(sys), port_label('input',1,'phi'), port_label('input',2,'the'), port_label('input',3,'psi'), port_label('input',4,'theta1'), port_label('input',5,'theta2'), port_label('input',6,'theta3'), port_label('output',1,'C_33')
  S-Function Builder1 : S-Function  InitFcn=try, set_param(gcb,'FunctionName','calc_C_11'), end  FunctionName=calc_C_11  SFunctionModules=calc_C_11_wrapper C_num_simp_11 C_num_simp_11_initialize C_num_simp_11_terminate  SFunctionDeploymentMode=off  EnableBusSupport=off  mask(S-Function Builder){}
      mask help: Simulink:masks:SFunctionBuilder_MD
      mask init: same as wrench_observer/Motion Equations with Manipulator /Inertia_Matrix/S-Function Builder
      settings: CopyFcn=set_param(gcbh,'LinkStatus','none')  PreSaveFcn=try, set_param(gcb,'FunctionName','calc_C_11'), end  OpenFcn=sfunctionwizard(gcbh)
      mask Display: plot(val(:,1),val(:,2)),disp(sys), port_label('input',1,'phi'), port_label('input',2,'the'), port_label('input',3,'psi'), port_label('input',4,'theta1'), port_label('input',5,'theta2'), port_label('input',6,'theta3'), port_label('output',1,'C_11')
  S-Function Builder2 : S-Function  InitFcn=try, set_param(gcb,'FunctionName','calc_C_12'), end  FunctionName=calc_C_12  SFunctionModules=calc_C_12_wrapper C_num_simp_12 C_num_simp_12_initialize C_num_simp_12_terminate  SFunctionDeploymentMode=off  EnableBusSupport=off  mask(S-Function Builder){}
      mask help: Simulink:masks:SFunctionBuilder_MD
      mask init: same as wrench_observer/Motion Equations with Manipulator /Inertia_Matrix/S-Function Builder
      settings: CopyFcn=set_param(gcbh,'LinkStatus','none')  PreSaveFcn=try, set_param(gcb,'FunctionName','calc_C_12'), end  OpenFcn=sfunctionwizard(gcbh)
      mask Display: plot(val(:,1),val(:,2)),disp(sys), port_label('input',1,'phi'), port_label('input',2,'the'), port_label('input',3,'psi'), port_label('input',4,'theta1'), port_label('input',5,'theta2'), port_label('input',6,'theta3'), port_label('output',1,'C_12')
  S-Function Builder3 : S-Function  InitFcn=try, set_param(gcb,'FunctionName','calc_C_13'), end  FunctionName=calc_C_13  SFunctionModules=calc_C_13_wrapper C_num_simp_13 C_num_simp_13_initialize C_num_simp_13_terminate  SFunctionDeploymentMode=off  EnableBusSupport=off  mask(S-Function Builder){}
      mask help: Simulink:masks:SFunctionBuilder_MD
      mask init: same as wrench_observer/Motion Equations with Manipulator /Inertia_Matrix/S-Function Builder
      settings: CopyFcn=set_param(gcbh,'LinkStatus','none')  PreSaveFcn=try, set_param(gcb,'FunctionName','calc_C_13'), end  OpenFcn=sfunctionwizard(gcbh)
      mask Display: plot(val(:,1),val(:,2)),disp(sys), port_label('input',1,'phi'), port_label('input',2,'the'), port_label('input',3,'psi'), port_label('input',4,'theta1'), port_label('input',5,'theta2'), port_label('input',6,'theta3'), port_label('output',1,'C_13')
  S-Function Builder4 : S-Function  InitFcn=try, set_param(gcb,'FunctionName','calc_C_21'), end  FunctionName=calc_C_21  SFunctionModules=calc_C_21_wrapper C_num_simp_21 C_num_simp_21_initialize C_num_simp_21_terminate  SFunctionDeploymentMode=off  EnableBusSupport=off  mask(S-Function Builder){}
      mask help: Simulink:masks:SFunctionBuilder_MD
      mask init: same as wrench_observer/Motion Equations with Manipulator /Inertia_Matrix/S-Function Builder
      settings: CopyFcn=set_param(gcbh,'LinkStatus','none')  PreSaveFcn=try, set_param(gcb,'FunctionName','calc_C_21'), end  OpenFcn=sfunctionwizard(gcbh)
      mask Display: plot(val(:,1),val(:,2)),disp(sys), port_label('input',1,'phi'), port_label('input',2,'the'), port_label('input',3,'psi'), port_label('input',4,'theta1'), port_label('input',5,'theta2'), port_label('input',6,'theta3'), port_label('output',1,'C_21')
  S-Function Builder5 : S-Function  InitFcn=try, set_param(gcb,'FunctionName','calc_C_22'), end  FunctionName=calc_C_22  SFunctionModules=calc_C_22_wrapper C_num_simp_22 C_num_simp_22_initialize C_num_simp_22_terminate rt_nonfinite rtGetInf rtGetNaN  SFunctionDeploymentMode=off  EnableBusSupport=off  mask(S-Function Builder){}
      mask help: Simulink:masks:SFunctionBuilder_MD
      mask init: same as wrench_observer/Motion Equations with Manipulator /Inertia_Matrix/S-Function Builder
      settings: CopyFcn=set_param(gcbh,'LinkStatus','none')  PreSaveFcn=try, set_param(gcb,'FunctionName','calc_C_22'), end  OpenFcn=sfunctionwizard(gcbh)
      mask Display: plot(val(:,1),val(:,2)),disp(sys), port_label('input',1,'phi'), port_label('input',2,'the'), port_label('input',3,'psi'), port_label('input',4,'theta1'), port_label('input',5,'theta2'), port_label('input',6,'theta3'), port_label('output',1,'C_22')
  S-Function Builder6 : S-Function  InitFcn=try, set_param(gcb,'FunctionName','calc_C_23'), end  FunctionName=calc_C_23  SFunctionModules=calc_C_23_wrapper C_num_simp_23 C_num_simp_23_initialize C_num_simp_23_terminate rt_nonfinite rtGetInf rtGetNaN  SFunctionDeploymentMode=off  EnableBusSupport=off  mask(S-Function Builder){}
      mask help: Simulink:masks:SFunctionBuilder_MD
      mask init: same as wrench_observer/Motion Equations with Manipulator /Inertia_Matrix/S-Function Builder
      settings: CopyFcn=set_param(gcbh,'LinkStatus','none')  PreSaveFcn=try, set_param(gcb,'FunctionName','calc_C_23'), end  OpenFcn=sfunctionwizard(gcbh)
      mask Display: plot(val(:,1),val(:,2)),disp(sys), port_label('input',1,'phi'), port_label('input',2,'the'), port_label('input',3,'psi'), port_label('input',4,'theta1'), port_label('input',5,'theta2'), port_label('input',6,'theta3'), port_label('output',1,'C_23')
  S-Function Builder7 : S-Function  InitFcn=try, set_param(gcb,'FunctionName','calc_C_31'), end  FunctionName=calc_C_31  SFunctionModules=calc_C_31_wrapper C_num_simp_31 C_num_simp_31_initialize C_num_simp_31_terminate  SFunctionDeploymentMode=off  EnableBusSupport=off  mask(S-Function Builder){}
      mask help: Simulink:masks:SFunctionBuilder_MD
      mask init: same as wrench_observer/Motion Equations with Manipulator /Inertia_Matrix/S-Function Builder
      settings: CopyFcn=set_param(gcbh,'LinkStatus','none')  PreSaveFcn=try, set_param(gcb,'FunctionName','calc_C_31'), end  OpenFcn=sfunctionwizard(gcbh)
      mask Display: plot(val(:,1),val(:,2)),disp(sys), port_label('input',1,'phi'), port_label('input',2,'the'), port_label('input',3,'psi'), port_label('input',4,'theta1'), port_label('input',5,'theta2'), port_label('input',6,'theta3'), port_label('output',1,'C_31')
  S-Function Builder8 : S-Function  InitFcn=try, set_param(gcb,'FunctionName','calc_C_32'), end  FunctionName=calc_C_32  SFunctionModules=calc_C_32_wrapper C_num_simp_32 C_num_simp_32_initialize C_num_simp_32_terminate rt_nonfinite rtGetInf rtGetNaN  SFunctionDeploymentMode=off  EnableBusSupport=off  mask(S-Function Builder){}
      mask help: Simulink:masks:SFunctionBuilder_MD
      mask init: same as wrench_observer/Motion Equations with Manipulator /Inertia_Matrix/S-Function Builder
      settings: CopyFcn=set_param(gcbh,'LinkStatus','none')  PreSaveFcn=try, set_param(gcb,'FunctionName','calc_C_32'), end  OpenFcn=sfunctionwizard(gcbh)
      mask Display: plot(val(:,1),val(:,2)),disp(sys), port_label('input',1,'phi'), port_label('input',2,'the'), port_label('input',3,'psi'), port_label('input',4,'theta1'), port_label('input',5,'theta2'), port_label('input',6,'theta3'), port_label('output',1,'C_32')
  C : Outport
  wires:
  S-Function Builder5/1 -> MATLAB Function/5(C22)
  theta2/1 -> S-Function Builder2/5, S-Function Builder3/5, S-Function Builder4/5, S-Function Builder5/5, S-Function Builder6/5, S-Function Builder7/5, S-Function Builder8/5, S-Function Builder/5, S-Function Builder1/5
  S-Function Builder3/1 -> MATLAB Function/3(C13)
  theta1/1 -> S-Function Builder2/4, S-Function Builder3/4, S-Function Builder4/4, S-Function Builder5/4, S-Function Builder6/4, S-Function Builder7/4, S-Function Builder8/4, S-Function Builder/4, S-Function Builder1/4
  theta3/1 -> S-Function Builder2/6, S-Function Builder3/6, S-Function Builder4/6, S-Function Builder5/6, S-Function Builder6/6, S-Function Builder7/6, S-Function Builder8/6, S-Function Builder/6, S-Function Builder1/6
  psi/1 -> S-Function Builder1/3, S-Function Builder2/3, S-Function Builder3/3, S-Function Builder4/3, S-Function Builder5/3, S-Function Builder6/3, S-Function Builder7/3, S-Function Builder8/3, S-Function Builder/3
  phi/1 -> S-Function Builder2/1, S-Function Builder3/1, S-Function Builder4/1, S-Function Builder5/1, S-Function Builder6/1, S-Function Builder7/1, S-Function Builder8/1, S-Function Builder/1, S-Function Builder1/1
  the/1 -> S-Function Builder2/2, S-Function Builder3/2, S-Function Builder4/2, S-Function Builder5/2, S-Function Builder6/2, S-Function Builder7/2, S-Function Builder8/2, S-Function Builder/2, S-Function Builder1/2
  S-Function Builder2/1 -> MATLAB Function/2(C12)
  S-Function Builder/1 -> MATLAB Function/9(C33)
  S-Function Builder7/1 -> MATLAB Function/7(C31)
  S-Function Builder1/1 -> MATLAB Function/1(C11)
  S-Function Builder8/1 -> MATLAB Function/8(C32)
  S-Function Builder6/1 -> MATLAB Function/6(C23)
  S-Function Builder4/1 -> MATLAB Function/4(C21)
  MATLAB Function/1(C) -> C/1
